simulink model "quadReduced"  (R2024a)
settings: Solver=VariableStepAuto  StartTime=0.0  StopTime=20  RelTol=1e-3
values from neighbouring files (symbols this model uses):
  A_x = 0.25    [playgrounMat.m]    (also in start.m; startEnglPaper.m; startReduced.m)
  A_y = 0.25    [playgrounMat.m]    (also in start.m; startEnglPaper.m; startReduced.m)
  A_z = 0.25    [playgrounMat.m]    (also in start.m; startEnglPaper.m; startReduced.m)
  b = 1.14 * 10^(-7)    (= 1.14e-07)    [start.m]    (also in startEnglPaper.m = 0.033)
  dt = 1e-4    (= 0.0001)    [start.m]    (also in startReduced.m)
  g = 9.81    [playgrounMat.m]    (also in start.m; startEnglPaper.m; startReduced.m)
  gamma_d = pi/3    (= 1.0471975512)    [start.m]    (also in startReduced.m = 0.2)
  I_r = 5.38 * 10 ^ (-5)    (= 5.38e-05)    [start.m]    (also in startEnglPaper.m = 3.38e-05; startReduced.m)
  I_x = 0.0151    [start.m]    (also in startEnglPaper.m = 0.004856; startReduced.m)
  I_y = 0.253    [start.m]    (also in startEnglPaper.m = 0.004856; startReduced.m = 0.0253)
  I_z = 0.0151    [start.m]    (also in startEnglPaper.m = 0.008801; startReduced.m)
  Icm = diag([Ix Iy Iz])    [start.m]    (also in startReduced.m)
  initial_quaternion = quaternion(initial_angles, 'euler', 'ZYX', 'frame')    [start.m]    (also in startReduced.m)
  k = 1.045 * 10^(-11)    (= 1.045e-11)    [start.m]    (also in startEnglPaper.m = 2.98e-06)
  K_gamma_D = 50    [start.m]    (also in startReduced.m = 0.14)
  K_gamma_D1 = K(1)    [playgrounMat.m]    (also in startReduced.m = 0.28992)
  K_gamma_I1 = K(3)    [playgrounMat.m]    (also in startReduced.m = 3.9584)
  K_gamma_P = 108    [start.m]    (also in startReduced.m = 0.35)
  K_gamma_P1 = K(2)    [playgrounMat.m]    (also in startReduced.m = 1.85548)
  K_psi_D = 40    [start.m]    (also in startEnglPaper.m = 9.6; startReduced.m = 0.24)
  K_psi_D1 = 0.0844    [startEnglPaper.m]    (also in startReduced.m = 0.4858)
  K_psi_I1 = 0    [startEnglPaper.m]    (also in startReduced.m = 6.6322)
  K_psi_P = 143    [start.m]    (also in startEnglPaper.m = 23.04; startReduced.m = 0.58)
  K_psi_P1 = 0.202    [startEnglPaper.m]    (also in startReduced.m = 3.11)
  K_theta_D = 58    [start.m]    (also in startEnglPaper.m = 9.6; startReduced.m = 0.14)
  K_theta_P = 141    [start.m]    (also in startEnglPaper.m = 23.04; startReduced.m = 0.35)
  K_y_D = 13.58    [start.m]    (also in startReduced.m)
  K_y_P = 33.18    [start.m]    (also in startReduced.m)
  l = 0.225    [start.m]    (also in startEnglPaper.m; startReduced.m)
  m = 1.44    [playgrounMat.m]    (also in start.m; startEnglPaper.m = 0.486; startReduced.m)
  m_s = [1/4 0 -1/(2*l) -1/(4*a_r); 1/4 -1/(2*l) 0 1/(4*a_r); 1/4 0 1/(2*l) -1/(4*a_r); 1/4 1/(2*l) 0 1/(4*a_r)]    [start.m]    (also in startReduced.m)
  omega_r = 1    [start.m]    (also in startReduced.m = 4)
  P_omega = diag([P_omega_x P_omega_y P_omega_z])    [start.m]    (also in startReduced.m)
  P_q = diag([P_q1 P_q2 P_q3])    [start.m]    (also in startReduced.m)
  psi_d = pi/5    (= 0.628318530718)    [start.m]    (also in startEnglPaper.m = 0.1; startReduced.m = 0.1)
  task_quaternion = quaternion(task_angles, 'euler', 'ZYX', 'frame')    [start.m]    (also in startReduced.m)
  theta_d = pi/4    (= 0.785398163397)    [start.m]    (also in startEnglPaper.m = -0.1; startReduced.m = -0.1)
  y_d = 100    [start.m]    (also in startReduced.m = 0.2)
undefined symbols (not defined in the file or in its folder): compact
libraries: slpidlib x4, aerolibutil x2, sharedtransform x1
(part 2 of 2)

== system quadReduced/quad_PID/PID regulator gamma ==
  gamma : Inport
  (gamma)' : Inport  Port=2
  Constant : Constant  Value=I_x
  Constant1 : Constant  Value=K_gamma_D1
  Constant2 : Constant  Value=gamma_d
  Constant3 : Constant  Value=K_gamma_I1
  Constant4 : Constant  Value=K_gamma_P1
  Constant5 : Constant  Value=gamma_d
  Derivative : Derivative
  Integrator : Integrator
  OnlyI : slpidlib/PID Controller  Controller=PID  Form=Parallel  TimeDomain=Continuous-time  UseExternalTs=off  SampleTime=-1  IntegratorMethod=Forward Euler  FilterMethod=Forward Euler  ControllerParametersSource=internal  P=0  I=K_gamma_D1  UseKiTs=off  D=0  UseExternalDerivativeSource=off  N=100  UseFilter=on  TunerSelectOption=Transfer Function Based (PID Tuner App)  InitialConditionSource=internal  InitialConditionForIntegrator=0  InitialConditionForFilter=0  DifferentiatorICPrevScaledInput=0  ExternalReset=none  TrackingMode=off  Kt=1  LimitOutput=off  SatLimitsSource=internal  UpperSaturationLimit=inf  LowerSaturationLimit=-inf  LinearizeAsGain=on  AntiWindupMode=none  Kb=1  LimitIntegrator=off  UpperIntegratorSaturationLimit=inf  LowerIntegratorSaturationLimit=-inf  POutMin=[]  POutMax=[]  IOutMin=[]  IOutMax=[]  DOutMin=[]  DOutMax=[]  NOutMin=[]  NOutMax=[]  SumOutMin=[]  SumOutMax=[]  SaturationOutMin=[]  SaturationOutMax=[]  PParamMin=[]  PParamMax=[]  IParamMin=[]  IParamMax=[]  DParamMin=[]  DParamMax=[]  NParamMin=[]  NParamMax=[]  KbParamMin=[]  KbParamMax=[]  KtParamMin=[]  KtParamMax=[]  KbOutMin=[]  KbOutMax=[]  KtOutMin=[]  KtOutMax=[]  IntegratorOutMin=[]  IntegratorOutMax=[]  FilterOutMin=[]  FilterOutMax=[]  SumI1OutMin=[]  SumI1OutMax=[]  SumI2OutMin=[]  SumI2OutMax=[]  SumI3OutMin=[]  SumI3OutMax=[]  SumI4OutMin=[]  SumI4OutMax=[]  SumDOutMin=[]  SumDOutMax=[]  DifferentiatorOutMin=[]  DifferentiatorOutMax=[]  FilterDiffOutCoefMin=[]  FilterDiffOutCoefMax=[]  ReciprocalOutMin=[]  ReciprocalOutMax=[]  SumDenOutMin=[]  SumDenOutMax=[]  SumNumOutMin=[]  SumNumOutMax=[]  DivideOutMin=[]  DivideOutMax=[]  UdiffTsProdOutMin=[]  UdiffTsProdOutMax=[]  NTsProdOutMin=[]  NTsProdOutMax=[]  UintegralTsProdOutMin=[]  UintegralTsProdOutMax=[]  UngainTsProdOutMin=[]  UngainTsProdOutMax=[]  ClampingZeroOutDataTypeStr=Inherit: Inherit via back propagation  ClampingZeroOutMin=[]  ClampingZeroOutMax=[]  FilterDenConstantOutDataTypeStr=Inherit: Inherit via back propagation  FilterDenConstantOutMin=[]  FilterDenConstantOutMax=[]  PCopyOutDataTypeStr=Inherit: Inherit via back propagation  PCopyOutMin=[]  PCopyOutMax=[]  NCopyOutDataTypeStr=Inherit: Inherit via back propagation  NCopyOutMin=[]  NCopyOutMax=[]  IntegratorContinuousStateAttributes=''  IntegratorStateMustResolveToSignalObject=off  IntegratorRTWStateStorageClass=Auto  FilterContinuousStateAttributes=''  FilterStateMustResolveToSignalObject=off  FilterRTWStateStorageClass=Auto  ParallelPVariant=InternalParameters  IdealPVariant=Disabled  IVariant=InternalParameters  DVariant=InternalParameters  IntegratorVariant=Continuous  SatVariant=Disabled  AWVariant=Passthrough  PCopyVariant=Disabled  TRVariant=Disabled  FdbkBlocksVariant=Forward  IdealPFdbkVariant=Disabled  SatFdbkVariant=Disabled  DerivativeFilterVariant=ContFilter  NVariant=InternalParameters  NCopyVariant=Disabled  FilterICVariant=InternalICsFilter  IntegratorICVariant=InternalICs  ExternalResetVariant=Disabled  TRSumVariant=Passthrough  SumFdbkVariant=Disabled  SumVariant=Sum_PID  TsampFilterVariant=InternalTs  TsampNgainVariant=Passthrough  TsampIntegralVariant=Disabled_SignalSpec  ExternalSaturationOutDataTypeStr=Inherit: Same as second input  DerivativeSourceVariant=ErrorSignal
  PID_coefs : slpidlib/PID Controller  Controller=PID  Form=Parallel  TimeDomain=Continuous-time  UseExternalTs=off  SampleTime=dt  IntegratorMethod=Forward Euler  FilterMethod=Forward Euler  ControllerParametersSource=internal  P=K_gamma_P1  I=K_gamma_I1  UseKiTs=off  D=K_gamma_D1  UseExternalDerivativeSource=off  N=100  UseFilter=on  TunerSelectOption=Transfer Function Based (PID Tuner App)  InitialConditionSource=internal  InitialConditionForIntegrator=0  InitialConditionForFilter=0  DifferentiatorICPrevScaledInput=0  ExternalReset=none  TrackingMode=off  Kt=1  LimitOutput=off  SatLimitsSource=internal  UpperSaturationLimit=inf  LowerSaturationLimit=-inf  LinearizeAsGain=on  AntiWindupMode=none  Kb=1  LimitIntegrator=off  UpperIntegratorSaturationLimit=inf  LowerIntegratorSaturationLimit=-inf  POutMin=[]  POutMax=[]  IOutMin=[]  IOutMax=[]  DOutMin=[]  DOutMax=[]  NOutMin=[]  NOutMax=[]  SumOutMin=[]  SumOutMax=[]  SaturationOutMin=[]  SaturationOutMax=[]  PParamMin=[]  PParamMax=[]  IParamMin=[]  IParamMax=[]  DParamMin=[]  DParamMax=[]  NParamMin=[]  NParamMax=[]  KbParamMin=[]  KbParamMax=[]  KtParamMin=[]  KtParamMax=[]  KbOutMin=[]  KbOutMax=[]  KtOutMin=[]  KtOutMax=[]  IntegratorOutMin=[]  IntegratorOutMax=[]  FilterOutMin=[]  FilterOutMax=[]  SumI1OutMin=[]  SumI1OutMax=[]  SumI2OutMin=[]  SumI2OutMax=[]  SumI3OutMin=[]  SumI3OutMax=[]  SumI4OutMin=[]  SumI4OutMax=[]  SumDOutMin=[]  SumDOutMax=[]  DifferentiatorOutMin=[]  DifferentiatorOutMax=[]  FilterDiffOutCoefMin=[]  FilterDiffOutCoefMax=[]  ReciprocalOutMin=[]  ReciprocalOutMax=[]  SumDenOutMin=[]  SumDenOutMax=[]  SumNumOutMin=[]  SumNumOutMax=[]  DivideOutMin=[]  DivideOutMax=[]  UdiffTsProdOutMin=[]  UdiffTsProdOutMax=[]  NTsProdOutMin=[]  NTsProdOutMax=[]  UintegralTsProdOutMin=[]  UintegralTsProdOutMax=[]  UngainTsProdOutMin=[]  UngainTsProdOutMax=[]  ClampingZeroOutDataTypeStr=Inherit: Inherit via back propagation  ClampingZeroOutMin=[]  ClampingZeroOutMax=[]  FilterDenConstantOutDataTypeStr=Inherit: Inherit via back propagation  FilterDenConstantOutMin=[]  FilterDenConstantOutMax=[]  PCopyOutDataTypeStr=Inherit: Inherit via back propagation  PCopyOutMin=[]  PCopyOutMax=[]  NCopyOutDataTypeStr=Inherit: Inherit via back propagation  NCopyOutMin=[]  NCopyOutMax=[]  IntegratorContinuousStateAttributes=''  IntegratorStateMustResolveToSignalObject=off  IntegratorRTWStateStorageClass=Auto  FilterContinuousStateAttributes=''  FilterStateMustResolveToSignalObject=off  FilterRTWStateStorageClass=Auto  ParallelPVariant=InternalParameters  IdealPVariant=Disabled  IVariant=InternalParameters  DVariant=InternalParameters  IntegratorVariant=Continuous  SatVariant=Disabled  AWVariant=Passthrough  PCopyVariant=Disabled  TRVariant=Disabled  FdbkBlocksVariant=Forward  IdealPFdbkVariant=Disabled  SatFdbkVariant=Disabled  DerivativeFilterVariant=ContFilter  NVariant=InternalParameters  NCopyVariant=Disabled  FilterICVariant=InternalICsFilter  IntegratorICVariant=InternalICs  ExternalResetVariant=Disabled  TRSumVariant=Passthrough  SumFdbkVariant=Disabled  SumVariant=Sum_PID  TsampFilterVariant=InternalTs  TsampNgainVariant=Passthrough  TsampIntegralVariant=Disabled_SignalSpec  ExternalSaturationOutDataTypeStr=Inherit: Same as second input  DerivativeSourceVariant=ErrorSignal
  Product{,1..3} (4 alike) : Product
  Sum : Sum  Inputs=+++|
  Sum1 : Sum  Inputs=|+-
  Sum2 : Sum  Inputs=|+-
  tau_gamma : Outport
  wires:
  Constant/1 -> Product2/2
  Product2/1 -> tau_gamma/1  "tau_gamma"
  Sum2/1 -> OnlyI/1, PID_coefs/1, Integrator/1, Product1/2
  (gamma)'/1 -> Sum1/2
  Constant2/1 -> Derivative/1
  Derivative/1 -> Sum1/1
  Constant5/1 -> Sum2/1
  gamma/1 -> Sum2/2
  Constant4/1 -> Product1/1
  Sum1/1 -> Product/2
  Product1/1 -> Sum/2
  Constant1/1 -> Product/1
  Product/1 -> Sum/1
  Integrator/1 -> Product3/2
  Constant3/1 -> Product3/1
  OnlyI/1 -> Sum/3
  PID_coefs/1 -> Product2/1

== system quadReduced/quad_PID/PID regulator psi ==
  psi : Inport
  (psi)' : Inport  Port=2
  Constant : Constant  Value=I_y
  Constant1 : Constant  Value=K_psi_D
  Constant2 : Constant  Value=psi_d
  Constant4 : Constant  Value=K_psi_P
  Constant5 : Constant  Value=psi_d
  Derivative : Derivative
  PID_coefs : slpidlib/PID Controller  Controller=PID  Form=Parallel  TimeDomain=Continuous-time  UseExternalTs=off  SampleTime=dt  IntegratorMethod=Forward Euler  FilterMethod=Forward Euler  ControllerParametersSource=internal  P=K_psi_P1  I=K_psi_I1  UseKiTs=off  D=K_psi_D1  UseExternalDerivativeSource=off  N=100  UseFilter=on  TunerSelectOption=Transfer Function Based (PID Tuner App)  InitialConditionSource=internal  InitialConditionForIntegrator=0  InitialConditionForFilter=0  DifferentiatorICPrevScaledInput=0  ExternalReset=none  TrackingMode=off  Kt=1  LimitOutput=off  SatLimitsSource=internal  UpperSaturationLimit=inf  LowerSaturationLimit=-inf  LinearizeAsGain=on  AntiWindupMode=none  Kb=1  LimitIntegrator=off  UpperIntegratorSaturationLimit=inf  LowerIntegratorSaturationLimit=-inf  POutMin=[]  POutMax=[]  IOutMin=[]  IOutMax=[]  DOutMin=[]  DOutMax=[]  NOutMin=[]  NOutMax=[]  SumOutMin=[]  SumOutMax=[]  SaturationOutMin=[]  SaturationOutMax=[]  PParamMin=[]  PParamMax=[]  IParamMin=[]  IParamMax=[]  DParamMin=[]  DParamMax=[]  NParamMin=[]  NParamMax=[]  KbParamMin=[]  KbParamMax=[]  KtParamMin=[]  KtParamMax=[]  KbOutMin=[]  KbOutMax=[]  KtOutMin=[]  KtOutMax=[]  IntegratorOutMin=[]  IntegratorOutMax=[]  FilterOutMin=[]  FilterOutMax=[]  SumI1OutMin=[]  SumI1OutMax=[]  SumI2OutMin=[]  SumI2OutMax=[]  SumI3OutMin=[]  SumI3OutMax=[]  SumI4OutMin=[]  SumI4OutMax=[]  SumDOutMin=[]  SumDOutMax=[]  DifferentiatorOutMin=[]  DifferentiatorOutMax=[]  FilterDiffOutCoefMin=[]  FilterDiffOutCoefMax=[]  ReciprocalOutMin=[]  ReciprocalOutMax=[]  SumDenOutMin=[]  SumDenOutMax=[]  SumNumOutMin=[]  SumNumOutMax=[]  DivideOutMin=[]  DivideOutMax=[]  UdiffTsProdOutMin=[]  UdiffTsProdOutMax=[]  NTsProdOutMin=[]  NTsProdOutMax=[]  UintegralTsProdOutMin=[]  UintegralTsProdOutMax=[]  UngainTsProdOutMin=[]  UngainTsProdOutMax=[]  ClampingZeroOutDataTypeStr=Inherit: Inherit via back propagation  ClampingZeroOutMin=[]  ClampingZeroOutMax=[]  FilterDenConstantOutDataTypeStr=Inherit: Inherit via back propagation  FilterDenConstantOutMin=[]  FilterDenConstantOutMax=[]  PCopyOutDataTypeStr=Inherit: Inherit via back propagation  PCopyOutMin=[]  PCopyOutMax=[]  NCopyOutDataTypeStr=Inherit: Inherit via back propagation  NCopyOutMin=[]  NCopyOutMax=[]  IntegratorContinuousStateAttributes=''  IntegratorStateMustResolveToSignalObject=off  IntegratorRTWStateStorageClass=Auto  FilterContinuousStateAttributes=''  FilterStateMustResolveToSignalObject=off  FilterRTWStateStorageClass=Auto  ParallelPVariant=InternalParameters  IdealPVariant=Disabled  IVariant=InternalParameters  DVariant=InternalParameters  IntegratorVariant=Continuous  SatVariant=Disabled  AWVariant=Passthrough  PCopyVariant=Disabled  TRVariant=Disabled  FdbkBlocksVariant=Forward  IdealPFdbkVariant=Disabled  SatFdbkVariant=Disabled  DerivativeFilterVariant=ContFilter  NVariant=InternalParameters  NCopyVariant=Disabled  FilterICVariant=InternalICsFilter  IntegratorICVariant=InternalICs  ExternalResetVariant=Disabled  TRSumVariant=Passthrough  SumFdbkVariant=Disabled  SumVariant=Sum_PID  TsampFilterVariant=InternalTs  TsampNgainVariant=Passthrough  TsampIntegralVariant=Disabled_SignalSpec  ExternalSaturationOutDataTypeStr=Inherit: Same as second input  DerivativeSourceVariant=ErrorSignal
  Product : Product
  Product1 : Product
  Product2 : Product
  Sum : Sum  Inputs=++|
  Sum1 : Sum  Inputs=|+-
  Sum2 : Sum  Inputs=|+-
  tau_psi : Outport
  wires:
  Constant/1 -> Product2/2
  Product2/1 -> tau_psi/1  "tau_psi"
  Sum2/1 -> PID_coefs/1, Product1/2
  (psi)'/1 -> Sum1/2
  Constant2/1 -> Derivative/1
  Derivative/1 -> Sum1/1
  Constant5/1 -> Sum2/1
  psi/1 -> Sum2/2
  Constant4/1 -> Product1/1
  Sum1/1 -> Product/2
  Product1/1 -> Sum/2
  Constant1/1 -> Product/1
  Product/1 -> Sum/1
  PID_coefs/1 -> Product2/1

== system quadReduced/quad_PID/PID regulator theta ==
  theta : Inport
  (theta)' : Inport  Port=2
  Constant : Constant  Value=I_z
  Constant1 : Constant  Value=K_theta_D
  Constant2 : Constant  Value=theta_d
  Constant4 : Constant  Value=K_theta_P
  Constant5 : Constant  Value=theta_d
  Derivative : Derivative
  PID_coefs : slpidlib/PID Controller  Controller=PID  Form=Parallel  TimeDomain=Continuous-time  UseExternalTs=off  SampleTime=dt  IntegratorMethod=Forward Euler  FilterMethod=Forward Euler  ControllerParametersSource=internal  P=K_gamma_P1  I=K_gamma_I1  UseKiTs=off  D=K_gamma_D1  UseExternalDerivativeSource=off  N=100  UseFilter=on  TunerSelectOption=Transfer Function Based (PID Tuner App)  InitialConditionSource=internal  InitialConditionForIntegrator=0  InitialConditionForFilter=0  DifferentiatorICPrevScaledInput=0  ExternalReset=none  TrackingMode=off  Kt=1  LimitOutput=off  SatLimitsSource=internal  UpperSaturationLimit=inf  LowerSaturationLimit=-inf  LinearizeAsGain=on  AntiWindupMode=none  Kb=1  LimitIntegrator=off  UpperIntegratorSaturationLimit=inf  LowerIntegratorSaturationLimit=-inf  POutMin=[]  POutMax=[]  IOutMin=[]  IOutMax=[]  DOutMin=[]  DOutMax=[]  NOutMin=[]  NOutMax=[]  SumOutMin=[]  SumOutMax=[]  SaturationOutMin=[]  SaturationOutMax=[]  PParamMin=[]  PParamMax=[]  IParamMin=[]  IParamMax=[]  DParamMin=[]  DParamMax=[]  NParamMin=[]  NParamMax=[]  KbParamMin=[]  KbParamMax=[]  KtParamMin=[]  KtParamMax=[]  KbOutMin=[]  KbOutMax=[]  KtOutMin=[]  KtOutMax=[]  IntegratorOutMin=[]  IntegratorOutMax=[]  FilterOutMin=[]  FilterOutMax=[]  SumI1OutMin=[]  SumI1OutMax=[]  SumI2OutMin=[]  SumI2OutMax=[]  SumI3OutMin=[]  SumI3OutMax=[]  SumI4OutMin=[]  SumI4OutMax=[]  SumDOutMin=[]  SumDOutMax=[]  DifferentiatorOutMin=[]  DifferentiatorOutMax=[]  FilterDiffOutCoefMin=[]  FilterDiffOutCoefMax=[]  ReciprocalOutMin=[]  ReciprocalOutMax=[]  SumDenOutMin=[]  SumDenOutMax=[]  SumNumOutMin=[]  SumNumOutMax=[]  DivideOutMin=[]  DivideOutMax=[]  UdiffTsProdOutMin=[]  UdiffTsProdOutMax=[]  NTsProdOutMin=[]  NTsProdOutMax=[]  UintegralTsProdOutMin=[]  UintegralTsProdOutMax=[]  UngainTsProdOutMin=[]  UngainTsProdOutMax=[]  ClampingZeroOutDataTypeStr=Inherit: Inherit via back propagation  ClampingZeroOutMin=[]  ClampingZeroOutMax=[]  FilterDenConstantOutDataTypeStr=Inherit: Inherit via back propagation  FilterDenConstantOutMin=[]  FilterDenConstantOutMax=[]  PCopyOutDataTypeStr=Inherit: Inherit via back propagation  PCopyOutMin=[]  PCopyOutMax=[]  NCopyOutDataTypeStr=Inherit: Inherit via back propagation  NCopyOutMin=[]  NCopyOutMax=[]  IntegratorContinuousStateAttributes=''  IntegratorStateMustResolveToSignalObject=off  IntegratorRTWStateStorageClass=Auto  FilterContinuousStateAttributes=''  FilterStateMustResolveToSignalObject=off  FilterRTWStateStorageClass=Auto  ParallelPVariant=InternalParameters  IdealPVariant=Disabled  IVariant=InternalParameters  DVariant=InternalParameters  IntegratorVariant=Continuous  SatVariant=Disabled  AWVariant=Passthrough  PCopyVariant=Disabled  TRVariant=Disabled  FdbkBlocksVariant=Forward  IdealPFdbkVariant=Disabled  SatFdbkVariant=Disabled  DerivativeFilterVariant=ContFilter  NVariant=InternalParameters  NCopyVariant=Disabled  FilterICVariant=InternalICsFilter  IntegratorICVariant=InternalICs  ExternalResetVariant=Disabled  TRSumVariant=Passthrough  SumFdbkVariant=Disabled  SumVariant=Sum_PID  TsampFilterVariant=InternalTs  TsampNgainVariant=Passthrough  TsampIntegralVariant=Disabled_SignalSpec  ExternalSaturationOutDataTypeStr=Inherit: Same as second input  DerivativeSourceVariant=ErrorSignal
  Product : Product
  Product1 : Product
  Product2 : Product
  Sum : Sum  Inputs=++|
  Sum1 : Sum  Inputs=|+-
  Sum2 : Sum  Inputs=|+-
  tau_theta : Outport
  wires:
  Constant/1 -> Product2/2
  Product2/1 -> tau_theta/1  "tau_theta"
  Sum2/1 -> PID_coefs/1, Product1/2
  (theta)'/1 -> Sum1/2
  Constant2/1 -> Derivative/1
  Derivative/1 -> Sum1/1
  Constant5/1 -> Sum2/1
  theta/1 -> Sum2/2
  Constant4/1 -> Product1/1
  Sum1/1 -> Product/2
  Product1/1 -> Sum/2
  Constant1/1 -> Product/1
  Product/1 -> Sum/1
  PID_coefs/1 -> Product2/1

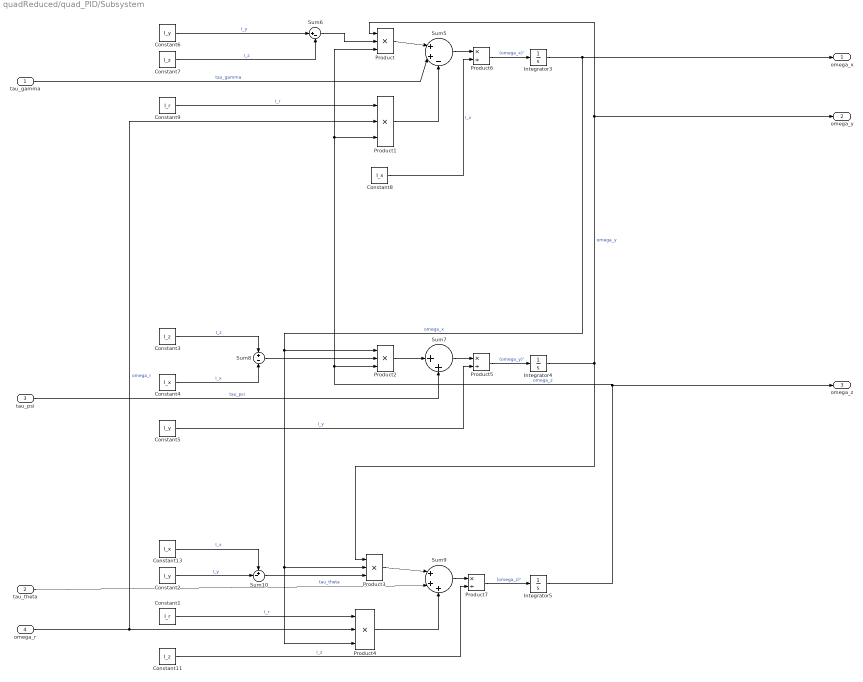
== system quadReduced/quad_PID/Subsystem ==
  tau_gamma : Inport
  tau_theta : Inport  Port=2
  tau_psi : Inport  Port=3
  omega_r : Inport  Port=4
  Constant1 : Constant  Value=I_r
  Constant11 : Constant  Value=I_z
  Constant13 : Constant  Value=I_x
  Constant2 : Constant  Value=I_y
  Constant3 : Constant  Value=I_z
  Constant4 : Constant  Value=I_x
  Constant5 : Constant  Value=I_y
  Constant6 : Constant  Value=I_y
  Constant7 : Constant  Value=I_z
  Constant8 : Constant  Value=I_x
  Constant9 : Constant  Value=I_r
  Integrator3 : Integrator
  Integrator4 : Integrator
  Integrator5 : Integrator
  Product{,1..4} (5 alike) : Product  Inputs=3
  Product5 : Product  Inputs=*/
  Product6 : Product  Inputs=*/
  Product7 : Product  Inputs=*/
  Sum10 : Sum  Inputs=+-|
  Sum5 : Sum  Inputs=|++-
  Sum6 : Sum  Inputs=|+-
  Sum7 : Sum  Inputs=|++
  Sum8 : Sum  Inputs=+|-
  Sum9 : Sum  Inputs=|+++
  omega_x : Outport
  omega_y : Outport  Port=2
  omega_z : Outport  Port=3
  wires:
  Constant11/1 -> Product7/2  "I_z"
  Constant8/1 -> Product6/2  "I_x"
  Constant5/1 -> Product5/2  "I_y"
  Constant4/1 -> Sum8/2  "I_x"
  Constant3/1 -> Sum8/1  "I_z"
  Constant2/1 -> Sum10/2  "I_y"
  Constant1/1 -> Product4/1  "I_r"
  tau_theta/1 -> Sum9/2  "tau_theta"
  tau_gamma/1 -> Sum5/2  "tau_gamma"
  Product7/1 -> Integrator5/1  "(omega_z)'"
  Product5/1 -> Integrator4/1  "(omega_y)'"
  Product4/1 -> Sum9/3
  Sum9/1 -> Product7/1
  Product3/1 -> Sum9/1
  Product6/1 -> Integrator3/1  "(omega_x)'"
  Sum6/1 -> Product/2
  Sum7/1 -> Product5/1
  Sum8/1 -> Product2/2
  Constant6/1 -> Sum6/1  "I_y"
  Constant9/1 -> Product1/1  "I_r"
  Sum5/1 -> Product6/1
  Product2/1 -> Sum7/1
  omega_r/1 -> Product1/2, Product4/2  "omega_r"
  Integrator4/1 -> Product3/1, Product/1, omega_y/1  "omega_y"
  Constant7/1 -> Sum6/2  "I_z"
  tau_psi/1 -> Sum7/2  "tau_psi"
  Sum10/1 -> Product3/3
  Product/1 -> Sum5/1
  Product1/1 -> Sum5/3
  Integrator3/1 -> Product2/1, Product3/2, Product4/3, omega_x/1  "omega_x"
  Constant13/1 -> Sum10/1  "I_x"
  Integrator5/1 -> omega_z/1, Product1/3, Product/3, Product2/3  "omega_z"

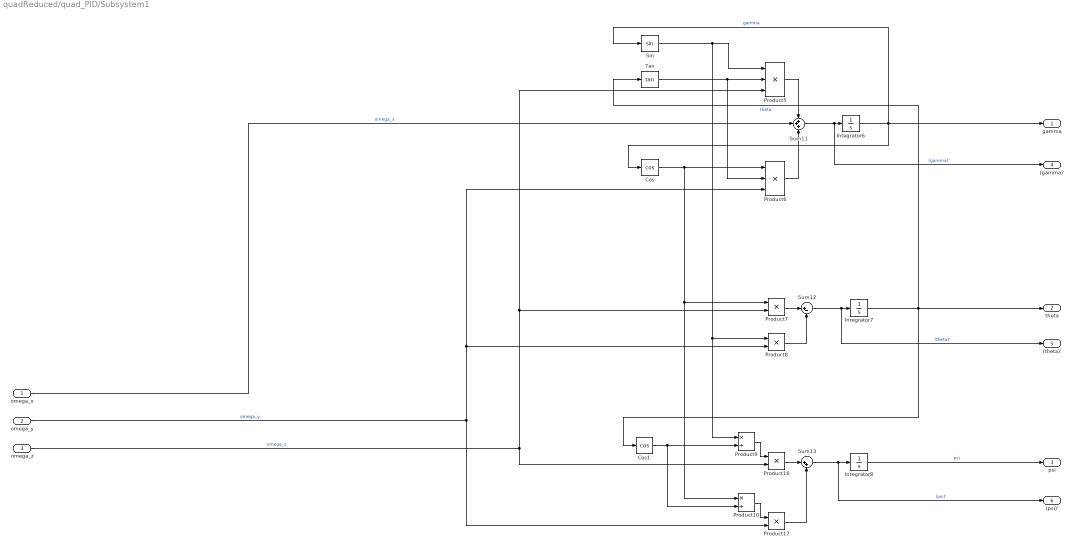
== system quadReduced/quad_PID/Subsystem1 ==
  omega_x : Inport
  omega_y : Inport  Port=2
  omega_z : Inport  Port=3
  Cos : Trigonometry  Operator=cos
  Cos1 : Trigonometry  Operator=cos
  Integrator6 : Integrator
  Integrator7 : Integrator
  Integrator8 : Integrator
  Product10 : Product  Inputs=*/
  Product{7..8,16..17} (4 alike) : Product
  Product5 : Product  Inputs=3
  Product6 : Product  Inputs=3
  Product9 : Product  Inputs=*/
  Sin : Trigonometry
  Sum11 : Sum  Inputs=+++
  Sum12 : Sum  Inputs=|+-
  Sum13 : Sum  Inputs=|++
  Tan : Trigonometry  Operator=tan
  gamma : Outport
  theta : Outport  Port=2
  psi : Outport  Port=3
  (gamma)' : Outport  Port=4
  (theta)' : Outport  Port=5
  (psi)' : Outport  Port=6
  wires:
  Product17/1 -> Sum13/2
  Product10/1 -> Product17/1
  Sum12/1 -> Integrator7/1, (theta)'/1  "(theta)'"
  Integrator8/1 -> psi/1  "psi"
  Product6/1 -> Sum11/3
  omega_y/1 -> Product17/2, Product8/2, Product6/3  "omega_y"
  omega_z/1 -> Product16/2, Product5/3, Product7/2  "omega_z"
  Cos/1 -> Product6/1, Product7/1, Product10/1
  Product7/1 -> Sum12/1
  Product8/1 -> Sum12/2
  Integrator6/1 -> Sin/1, gamma/1, Cos/1  "gamma"
  Product5/1 -> Sum11/1
  Integrator7/1 -> Cos1/1, Tan/1, theta/1  "theta"
  Product16/1 -> Sum13/1
  Cos1/1 -> Product9/2, Product10/2
  Sin/1 -> Product5/1, Product8/1, Product9/1
  Sum11/1 -> Integrator6/1, (gamma)'/1  "(gamma)'"
  Tan/1 -> Product6/2, Product5/2
  omega_x/1 -> Sum11/2  "omega_x"
  Sum13/1 -> Integrator8/1, (psi)'/1  "(psi)'"
  Product9/1 -> Product16/1

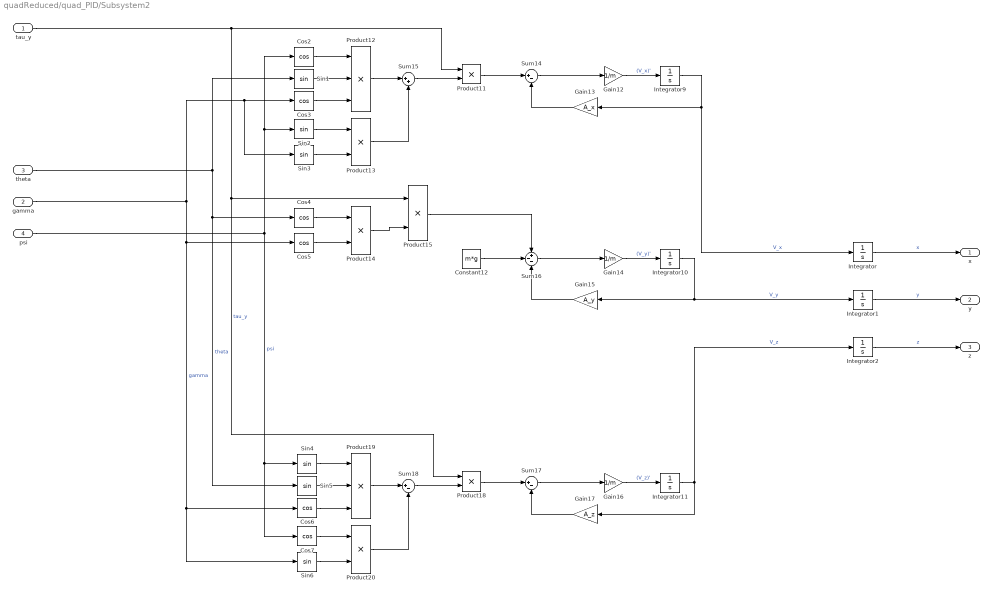
== system quadReduced/quad_PID/Subsystem2 ==
  tau_y : Inport
  gamma : Inport  Port=2
  theta : Inport  Port=3
  psi : Inport  Port=4
  Constant12 : Constant  Value=m*g
  Cos{2..7} (6 alike) : Trigonometry  Operator=cos
  Gain12 : Gain  Gain=1/m
  Gain13 : Gain  Gain=A_x
  Gain14 : Gain  Gain=1/m
  Gain15 : Gain  Gain=A_y
  Gain16 : Gain  Gain=1/m
  Gain17 : Gain  Gain=A_z
  Integrator{,1..2,9..11} (6 alike) : Integrator
  Product{11,13..15,18,20} (6 alike) : Product
  Product12 : Product  Inputs=3
  Product19 : Product  Inputs=3
  Sin{1..6} (6 alike) : Trigonometry
  Sum14 : Sum  Inputs=|+-
  Sum15 : Sum  Inputs=|++
  Sum16 : Sum  Inputs=+--
  Sum17 : Sum  Inputs=|+-
  Sum18 : Sum  Inputs=|+-
  x : Outport
  y : Outport  Port=2
  z : Outport  Port=3
  wires:
  Integrator2/1 -> z/1  "z"
  Integrator1/1 -> y/1  "y"
  Integrator/1 -> x/1  "x"
  Sin5/1 -> Product19/2
  Cos6/1 -> Product19/3
  Sum17/1 -> Gain16/1
  Sum18/1 -> Product18/2
  Gain13/1 -> Sum14/2
  Sin2/1 -> Product13/1
  Product18/1 -> Sum17/1
  Sum14/1 -> Gain12/1
  Product13/1 -> Sum15/2
  Sum15/1 -> Product11/2
  Sin1/1 -> Product12/2
  Product12/1 -> Sum15/1
  Integrator10/1 -> Gain15/1, Integrator1/1  "V_y"
  Sum16/1 -> Gain14/1
  Gain15/1 -> Sum16/3
  Sin3/1 -> Product13/2
  Gain17/1 -> Sum17/2
  Cos7/1 -> Product20/1
  Constant12/1 -> Sum16/2
  Gain14/1 -> Integrator10/1  "(V_y)'"
  Product19/1 -> Sum18/1
  Product20/1 -> Sum18/2
  Integrator9/1 -> Gain13/1, Integrator/1  "V_x"
  theta/1 -> Sin1/1, Cos4/1, Sin5/1  "theta"
  gamma/1 -> Cos3/1, Sin3/1, Cos5/1, Cos6/1, Sin6/1  "gamma"
  Product14/1 -> Product15/2
  tau_y/1 -> Product11/1, Product15/1, Product18/1  "tau_y"
  Cos2/1 -> Product12/1
  Gain16/1 -> Integrator11/1  "(V_z)'"
  Gain12/1 -> Integrator9/1  "(V_x)'"
  Cos3/1 -> Product12/3
  Integrator11/1 -> Integrator2/1, Gain17/1  "V_z"
  Sin6/1 -> Product20/2
  Sin4/1 -> Product19/1
  Product11/1 -> Sum14/1
  Cos5/1 -> Product14/2
  psi/1 -> Sin2/1, Cos2/1, Sin4/1, Cos7/1  "psi"
  Product15/1 -> Sum16/1
  Cos4/1 -> Product14/1

== system quadReduced/quad_PID/Subsystem3 ==
  omega_1 : Inport
  omega_2 : Inport  Port=2
  omega_3 : Inport  Port=3
  omega_4 : Inport  Port=4
  Gain1 : Gain  Gain=l*k
  Gain2 : Gain  Gain=l*k
  Gain3 : Gain  Gain=b
  Gain4 : Gain  Gain=k
  Math Function{,1..5} (6 alike) : Math  Operator=square  SignedPower=on
  Mux : Mux
  Mux1 : Mux
  Sum of Elements : Sum  Inputs=+
  Sum of Elements1 : Sum  Inputs=+
  Sum1 : Sum  Inputs=|-+
  Sum2 : Sum  Inputs=|-+
  tau_gamma : Outport
  tau_theta : Outport  Port=2
  tau_psi : Outport  Port=3
  tau_y : Outport  Port=4
  wires:
  omega_4/1 -> Math Function1/1, Mux/4, Mux1/4
  omega_1/1 -> Mux/1, Mux1/1, Math Function2/1
  omega_3/1 -> Mux/3, Mux1/3, Math Function3/1
  omega_2/1 -> Math Function/1, Mux/2, Mux1/2
  Mux1/1 -> Math Function5/1
  Math Function5/1 -> Gain4/1
  Gain4/1 -> Sum of Elements1/1
  Sum of Elements1/1 -> tau_y/1
  Sum of Elements/1 -> tau_psi/1
  Gain3/1 -> Sum of Elements/1
  Math Function4/1 -> Gain3/1
  Mux/1 -> Math Function4/1
  Math Function3/1 -> Sum2/2
  Math Function2/1 -> Sum2/1
  Math Function1/1 -> Sum1/2
  Math Function/1 -> Sum1/1
  Gain2/1 -> tau_gamma/1
  Sum1/1 -> Gain2/1
  Sum2/1 -> Gain1/1
  Gain1/1 -> tau_theta/1

== system quadReduced/quad_PID/Subsystem4 ==
  omega_1 : Inport
  omega_2 : Inport  Port=2
  omega_3 : Inport  Port=3
  omega_4 : Inport  Port=4
  Gain1 : Gain  Gain=l*k
  Gain2 : Gain  Gain=l*k
  Gain3 : Gain  Gain=b
  Gain4 : Gain  Gain=k
  Math Function{,1..5} (6 alike) : Math  Operator=square  SignedPower=on
  Mux : Mux
  Mux1 : Mux
  Sum of Elements : Sum  Inputs=+
  Sum of Elements1 : Sum  Inputs=+
  Sum1 : Sum  Inputs=|-+
  Sum2 : Sum  Inputs=|-+
  tau_gamma : Outport
  tau_theta : Outport  Port=2
  tau_psi : Outport  Port=3
  tau_y : Outport  Port=4
  wires:
  omega_4/1 -> Math Function1/1, Mux/4, Mux1/4
  omega_1/1 -> Mux/1, Mux1/1, Math Function2/1
  omega_3/1 -> Mux/3, Mux1/3, Math Function3/1
  omega_2/1 -> Math Function/1, Mux/2, Mux1/2
  Mux1/1 -> Math Function5/1
  Math Function5/1 -> Gain4/1
  Gain4/1 -> Sum of Elements1/1
  Sum of Elements1/1 -> tau_y/1
  Sum of Elements/1 -> tau_psi/1
  Gain3/1 -> Sum of Elements/1
  Math Function4/1 -> Gain3/1
  Mux/1 -> Math Function4/1
  Math Function3/1 -> Sum2/2
  Math Function2/1 -> Sum2/1
  Math Function1/1 -> Sum1/2
  Math Function/1 -> Sum1/1
  Gain2/1 -> tau_gamma/1
  Sum1/1 -> Gain2/1
  Sum2/1 -> Gain1/1
  Gain1/1 -> tau_theta/1

== system quadReduced/quad_quaternion/ Сonjugate of the estimated quaternion (q*_m) ==
  q0_m : Inport
  q1_m : Inport  Port=2
  q2_m : Inport  Port=3
  q3_m : Inport  Port=4
  Constant2 : Constant  Value=-1
  Product11 : Product
  Product12 : Product
  Product13 : Product
  Conj(q0_m) : Outport
  Conj(q1_m) : Outport  Port=2
  Conj(q2_m) : Outport  Port=3
  Conj(q3_m) : Outport  Port=4
  wires:
  q0_m/1 -> Conj(q0_m)/1
  Product11/1 -> Conj(q1_m)/1
  Product12/1 -> Conj(q2_m)/1
  Constant2/1 -> Product13/2, Product11/2, Product12/2
  q3_m/1 -> Product13/1
  q2_m/1 -> Product12/1
  Product13/1 -> Conj(q3_m)/1
  q1_m/1 -> Product11/1

== system quadReduced/quad_quaternion/PD regulator draft ==
  y : Inport
  gamma : Inport  Port=2
  theta : Inport  Port=3
  Constant : Constant  Value=g
  Constant1 : Constant  Value=K_y_D
  Constant2 : Constant  Value=y_d
  Constant4 : Constant  Value=K_y_P
  Constant5 : Constant  Value=y_d
  Constant7 : Constant  Value=m
  Cos : Trigonometry  Operator=cos
  Cos1 : Trigonometry  Operator=cos
  Derivative : Derivative
  Derivative1 : Derivative
  Product{,1,3..4} (4 alike) : Product
  Product2 : Product  Inputs=*/
  Sum : Sum  Inputs=+++
  Sum1 : Sum  Inputs=|+-
  Sum2 : Sum  Inputs=|+-
  tau_y : Outport
  wires:
  Cos/1 -> Product3/1
  Product/1 -> Sum/1
  Constant1/1 -> Product/1
  Product1/1 -> Sum/3
  Sum1/1 -> Product/2
  Constant4/1 -> Product1/1
  Constant2/1 -> Derivative/1
  y/1 -> Sum2/2, Derivative1/1  "y"
  Derivative1/1 -> Sum1/2
  Constant/1 -> Sum/2
  Derivative/1 -> Sum1/1
  Constant5/1 -> Sum2/1
  Product3/1 -> Product2/2
  Constant7/1 -> Product2/1
  Cos1/1 -> Product3/2
  Sum2/1 -> Product1/2
  theta/1 -> Cos1/1  "theta"
  gamma/1 -> Cos/1  "gamma"
  Sum/1 -> Product4/1
  Product4/1 -> tau_y/1  "tau_y"
  Product2/1 -> Product4/2

== system quadReduced/quad_quaternion/Quadtoror dynamic ==
  tau : Inport
  Constant : Constant  Value=0
  Gain : Gain  Gain=Icm  Multiplication=Matrix(K*u) (u vector)
  Gain1 : Gain  Gain=inv(Icm)  Multiplication=Matrix(K*u) (u vector)
  Gain2 : Gain  Gain=inv(Icm)  Multiplication=Matrix(K*u) (u vector)
  Gain3 : Gain  Gain=-0.5
  Mux : Mux  Inputs=2
  Product : Product
  Quaternion Multiplication : aerolibutil/Quaternion Multiplication
  Sum : Sum  Inputs=|-+
  omegas : Integrator
  quaternion : Integrator  InitialCondition=compact(initial_quaternion)'
  q : Outport
  omega : Outport  Port=2
  wires:
  Product/1 -> Gain1/1
  omegas/1 -> omega/1, [omega], Mux/2
  tau/1 -> Gain2/1
  Gain1/1 -> Sum/1
  Gain2/1 -> Sum/2
  Sum/1 -> omegas/1
  Constant/1 -> Mux/1
  Mux/1 -> Quaternion Multiplication/1
  Quaternion Multiplication/1 -> Gain3/1
  quaternion/1 -> q/1, Quaternion Multiplication/2
  [omega] -> Product/1, Gain/1
  Gain/1 -> Product/2
  Gain3/1 -> quaternion/1

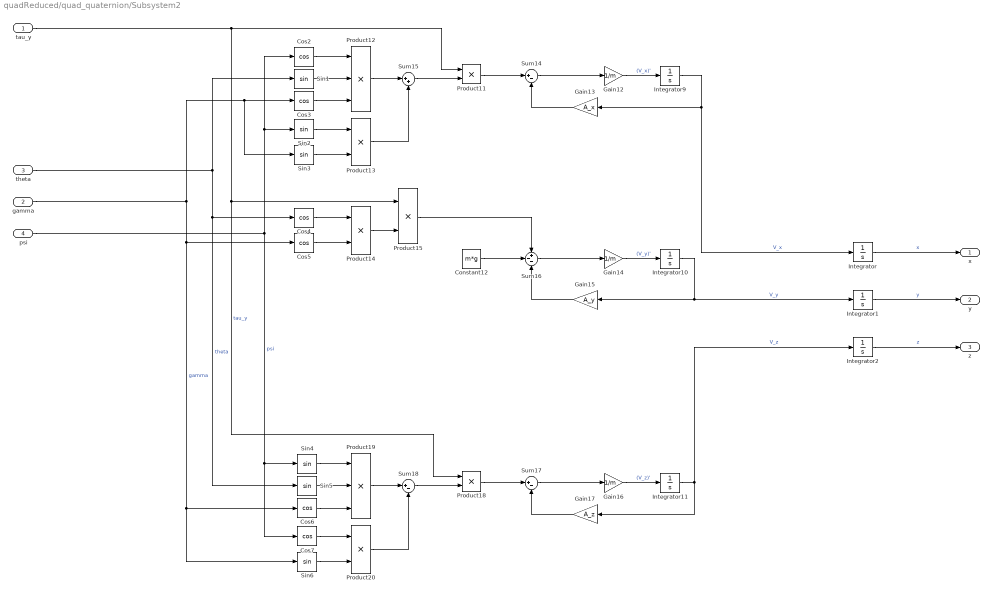
== system quadReduced/quad_quaternion/Subsystem2 ==
  tau_y : Inport
  gamma : Inport  Port=2
  theta : Inport  Port=3
  psi : Inport  Port=4
  Constant12 : Constant  Value=m*g
  Cos{2..7} (6 alike) : Trigonometry  Operator=cos
  Gain12 : Gain  Gain=1/m
  Gain13 : Gain  Gain=A_x
  Gain14 : Gain  Gain=1/m
  Gain15 : Gain  Gain=A_y
  Gain16 : Gain  Gain=1/m
  Gain17 : Gain  Gain=A_z
  Integrator{,1..2,9..11} (6 alike) : Integrator
  Product{11,13..15,18,20} (6 alike) : Product
  Product12 : Product  Inputs=3
  Product19 : Product  Inputs=3
  Sin{1..6} (6 alike) : Trigonometry
  Sum14 : Sum  Inputs=|+-
  Sum15 : Sum  Inputs=|++
  Sum16 : Sum  Inputs=+--
  Sum17 : Sum  Inputs=|+-
  Sum18 : Sum  Inputs=|+-
  x : Outport
  y : Outport  Port=2
  z : Outport  Port=3
  wires:
  Cos4/1 -> Product14/1
  Product15/1 -> Sum16/1
  psi/1 -> Cos7/1, Sin4/1, Cos2/1, Sin2/1  "psi"
  Cos5/1 -> Product14/2
  Product11/1 -> Sum14/1
  Sin4/1 -> Product19/1
  Sin6/1 -> Product20/2
  Integrator11/1 -> Gain17/1, Integrator2/1  "V_z"
  Cos3/1 -> Product12/3
  Gain12/1 -> Integrator9/1  "(V_x)'"
  Gain16/1 -> Integrator11/1  "(V_z)'"
  Cos2/1 -> Product12/1
  tau_y/1 -> Product18/1, Product15/1, Product11/1  "tau_y"
  Product14/1 -> Product15/2
  gamma/1 -> Sin6/1, Cos6/1, Cos5/1, Sin3/1, Cos3/1  "gamma"
  theta/1 -> Sin5/1, Cos4/1, Sin1/1  "theta"
  Integrator9/1 -> Integrator/1, Gain13/1  "V_x"
  Product20/1 -> Sum18/2
  Product19/1 -> Sum18/1
  Gain14/1 -> Integrator10/1  "(V_y)'"
  Constant12/1 -> Sum16/2
  Cos7/1 -> Product20/1
  Gain17/1 -> Sum17/2
  Sin3/1 -> Product13/2
  Gain15/1 -> Sum16/3
  Sum16/1 -> Gain14/1
  Integrator10/1 -> Integrator1/1, Gain15/1  "V_y"
  Product12/1 -> Sum15/1
  Sin1/1 -> Product12/2
  Sum15/1 -> Product11/2
  Product13/1 -> Sum15/2
  Sum14/1 -> Gain12/1
  Product18/1 -> Sum17/1
  Sin2/1 -> Product13/1
  Gain13/1 -> Sum14/2
  Sum18/1 -> Product18/2
  Sum17/1 -> Gain16/1
  Cos6/1 -> Product19/3
  Sin5/1 -> Product19/2
  Integrator/1 -> x/1  "x"
  Integrator1/1 -> y/1  "y"
  Integrator2/1 -> z/1  "z"

== system quadReduced/quad_quaternion/Subsystem4 ==
  omega_1 : Inport
  omega_2 : Inport  Port=2
  omega_3 : Inport  Port=3
  omega_4 : Inport  Port=4
  Gain1 : Gain  Gain=l*k
  Gain2 : Gain  Gain=l*k
  Gain3 : Gain  Gain=b
  Gain4 : Gain  Gain=k
  Math Function{,1..5} (6 alike) : Math  Operator=square  SignedPower=on
  Mux : Mux
  Mux1 : Mux
  Sum of Elements : Sum  Inputs=+
  Sum of Elements1 : Sum  Inputs=+
  Sum1 : Sum  Inputs=|-+
  Sum2 : Sum  Inputs=|-+
  tau_gamma : Outport
  tau_theta : Outport  Port=2
  tau_psi : Outport  Port=3
  tau_y : Outport  Port=4
  wires:
  Gain1/1 -> tau_theta/1
  Sum2/1 -> Gain1/1
  Sum1/1 -> Gain2/1
  Gain2/1 -> tau_gamma/1
  Math Function/1 -> Sum1/1
  Math Function1/1 -> Sum1/2
  Math Function2/1 -> Sum2/1
  Math Function3/1 -> Sum2/2
  Mux/1 -> Math Function4/1
  Math Function4/1 -> Gain3/1
  Gain3/1 -> Sum of Elements/1
  Sum of Elements/1 -> tau_psi/1
  Sum of Elements1/1 -> tau_y/1
  Gain4/1 -> Sum of Elements1/1
  Math Function5/1 -> Gain4/1
  Mux1/1 -> Math Function5/1
  omega_2/1 -> Mux1/2, Mux/2, Math Function/1
  omega_3/1 -> Math Function3/1, Mux1/3, Mux/3
  omega_1/1 -> Math Function2/1, Mux1/1, Mux/1
  omega_4/1 -> Mux1/4, Mux/4, Math Function1/1

== matlab function quadReduced/quad_PID/MATLAB Function ==
  data: tau_y input; omega_1 output; omega_2 output; omega_3 output; omega_4 output; tau_gamma input; tau_theta input; tau_psi input; k input; l input; b input
function [omega_1,omega_2,omega_3,omega_4] = fcn(tau_y,tau_gamma,tau_theta,tau_psi,k,l,b)
omega_1 = tau_y/(4*k) - tau_theta/(2*k*l) - tau_psi/(4*b);
omega_2 = tau_y/(4*k) - tau_gamma/(2*k*l) + tau_psi/(4*b);
omega_3 = tau_y/(4*k) + tau_theta/(2*k*l) - tau_psi/(4*b);
omega_4 = tau_y/(4*k) + tau_gamma/(2*k*l) + tau_psi/(4*b);

== matlab function quadReduced/quad_PD/MATLAB Function ==
  data: tau_y input; omega_1 output; omega_2 output; omega_3 output; omega_4 output; tau_gamma input; tau_theta input; tau_psi input; k input; l input; b input
function [omega_1,omega_2,omega_3,omega_4] = fcn(tau_y,tau_gamma,tau_theta,tau_psi,k,l,b)
omega_1 = tau_y/(4*k) - tau_theta/(2*k*l) - tau_psi/(4*b);
omega_2 = tau_y/(4*k) - tau_gamma/(2*k*l) + tau_psi/(4*b);
omega_3 = tau_y/(4*k) + tau_theta/(2*k*l) - tau_psi/(4*b);
omega_4 = tau_y/(4*k) + tau_gamma/(2*k*l) + tau_psi/(4*b);

== matlab function quadReduced/quad_PD_linear/MATLAB Function ==
  data: tau_y input; omega_1 output; omega_2 output; omega_3 output; omega_4 output; tau_gamma input; tau_theta input; tau_psi input; k input; l input; b input
function [omega_1,omega_2,omega_3,omega_4] = fcn(tau_y,tau_gamma,tau_theta,tau_psi,k,l,b)
omega_1 = tau_y/(4*k) - tau_theta/(2*k*l) - tau_psi/(4*b);
omega_2 = tau_y/(4*k) - tau_gamma/(2*k*l) + tau_psi/(4*b);
omega_3 = tau_y/(4*k) + tau_theta/(2*k*l) - tau_psi/(4*b);
omega_4 = tau_y/(4*k) + tau_gamma/(2*k*l) + tau_psi/(4*b);
